simulink library "FireflySimLib"  (R2018a)
settings: Solver=VariableStepAuto  StartTime=0.0  StopTime=10.0  RelTol=1e-3
values from neighbouring files (symbols this model uses):
  mass = parmodel.mass    [LowLevelGeometricController.m]
  p = [ -lengthsoccerfield(1)/2*(yi-centersoccerfieldpic(2))/centersoccerfieldpic(2) lengthsoccerfield(2)/2*(xi-centersoccerfieldpic(1))/centersoccerfieldpic(2)]    [clicks2traj.m]    (also in lqrtrajgeneration.m = size(M,1))
  T = Tlowerlimit    [LowLevelGeometricController.m]    (also in T.mat = ; lqrtrajgeneration.m = T-T(1))
undefined symbols (not defined in the file or in its folder): cdrag, g, lambda, mat2cell, omega, parcontroller, pose0, v
libraries: vrlib x5, sharedtransform x3, dspindex x1, dspsigattribs x1, shared6dof x1
settings Model: Creator=duarteantunes  LastModifiedBy=duarteantunes

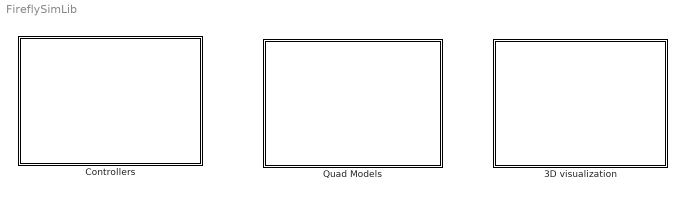
== system FireflySimLib ==
  3D visualization : Subsystem
      mask Display: image('/Users/duarteantunes/surfdrive/AssistantProfessor/Software/Matlab/Firefly/tests/FirstProject/RobotLove/Aux/showpic.png');
  Controllers : Subsystem
      mask Display: image('/Users/duarteantunes/surfdrive/AssistantProfessor/Software/Matlab/Firefly/tests/FirstProject/RobotLove/Aux/pid.png');
  Quad Models : Subsystem
      mask Display: image('/Users/duarteantunes/surfdrive/AssistantProfessor/Software/Matlab/Firefly/tests/FirstProject/RobotLove/Aux/drone.jpg');

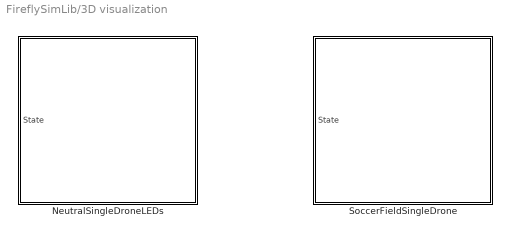
== system FireflySimLib/3D visualization ==
  NeutralSingleDroneLEDs : Subsystem
  SoccerFieldSingleDrone : Subsystem  AncestorBlock=FireflyLib/3D visualization/NeutralSingleDroneLEDs

== system FireflySimLib/Controllers ==
  Controller : Subsystem

== system FireflySimLib/Quad Models ==
  Quad rigid body model : Subsystem

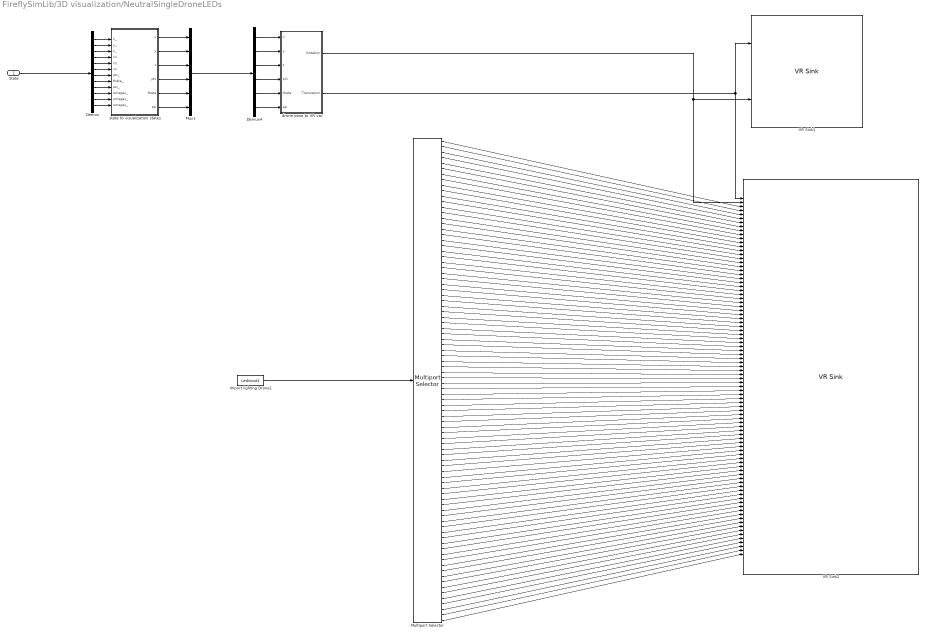
== system FireflySimLib/3D visualization/NeutralSingleDroneLEDs ==
  State : Inport
  Demux : Demux  Outputs=12
  Demux4 : Demux  Outputs=6
  Import lighting Drone1 : FromWorkspace  VariableName=Ledinput1  SampleTime=0
  Multiport Selector : dspindex/Multiport Selector  rowsOrCols=Rows  idxCellArray=mat2cell([1:88],1,ones(88,1))  idxErrMode=Clip Index
  Mux1 : Mux  Inputs=6
  VR Sink1 : vrlib/VR Sink  InstantiateOnLoad=on  SampleTime=0.1  ViewEnable=on  RemoteChange=off  RemoteView=off  FieldsWritten=Quad1.translation.3.1.1.double#Quad1.rotation.4.1.1.double  WorldFileName=SoccerFieldSingleDrone.wrl  AutoView=off  VideoDimensions=[]  AllowVariableSize=off
      settings: SourceProductBaseCode=VR
  VR Sink2 : vrlib/VR Sink  InstantiateOnLoad=on  SampleTime=0.1  ViewEnable=on  RemoteChange=off  RemoteView=off  FieldsWritten=Quad1.translation.3.1.1.double#Quad1.rotation.4.1.1.double#led1_1.emissiveColor.3.1.1.double#led1_2.emissiveColor.3.1.1.double#led1_3.emissiveColor.3.1.1.double#led1_4.emissiveColor.3.1.1.double#led1_5.emissiveColor.3.1.1.double#led1_6.emissiveColor.3.1.1.double#led1_7.emissiveColor.3.1.1.double#led1_8.emissiveColor.3.1.1.double#led1_9.emissiveColor.3.1.1.double#led1_10.emissiveColor.3.1.1.double#led1_11.emissiveColor.3.1.1.double#led1_12.emissiveColor.3.1.1.double#led1_13.emissiveColor.3.1.1.double#led1_14.emissiveColor.3.1.1.double#led1_15.emissiveColor.3.1.1.double#led1_16.emissiveColor.3.1.1.double#led1_17.emissiveColor.3.1.1.double#led1_18.emissiveColor.3.1.1.double#led1_19.emissiveColor.3.1.1.double#led1_20.emissiveColor.3.1.1.double#led1_21.emissiveColor.3.1.1.double#led1_22.emissiveColor.3.1.1.double#led1_23.emissiveColor.3.1.1.double#led1_24.emissiveColor.3.1.1.double#led1_25.emissiveColor.3.1.1.double#led1_26.emissiveColor.3.1.1.double#led1_27.emissiveColor.3.1.1.double#led1_28.emissiveColor.3.1.1.double#led1_29.emissiveColor.3.1.1.double#led1_30.emissiveColor.3.1.1.double#led1_31.emissiveColor.3.1.1.double#led1_32.emissiveColor.3.1.1.double#led1_33.emissiveColor.3.1.1.double#led1_34.emissiveColor.3.1.1.double#led1_35.emissiveColor.3.1.1.double#led1_36.emissiveColor.3.1.1.double#led1_37.emissiveColor.3.1.1.double#led1_38.emissiveColor.3.1.1.double#led1_39.emissiveColor.3.1.1.double#led1_40.emissiveColor.3.1.1.double#led1_41.emissiveColor.3.1.1.double#led1_42.emissiveColor.3.1.1.double#led1_43.emissiveColor.3.1.1.double#led1_44.emissiveColor.3.1.1.double#led1_45.emissiveColor.3.1.1.double#led1_46.emissiveColor.3.1.1.double#led1_47.emissiveColor.3.1.1.double#led1_48.emissiveColor.3.1.1.double#led1_49.emissiveColor.3.1.1.double#led1_50.emissiveColor.3.1.1.double#led1_51.emissiveColor.3.1.1.double#led1_52.emissiveColor.3.1.1.double#led1_53.emissiveColor.3.1.1.double#led1_54.emissiveColor.3.1.1.double#led1_55.emissiveColor.3.1.1.double#led1_56.emissiveColor.3.1.1.double#led1_57.emissiveColor.3.1.1.double#led1_58.emissiveColor.3.1.1.double#led1_59.emissiveColor.3.1.1.double#led1_60.emissiveColor.3.1.1.double#led1_61.emissiveColor.3.1.1.double#led1_62.emissiveColor.3.1.1.double#led1_63.emissiveColor.3.1.1.double#led1_64.emissiveColor.3.1.1.double#led1_65.emissiveColor.3.1.1.double#led1_66.emissiveColor.3.1.1.double#led1_67.emissiveColor.3.1.1.double#led1_68.emissiveColor.3.1.1.double#led1_69.emissiveColor.3.1.1.double#led1_70.emissiveColor.3.1.1.double#led1_71.emissiveColor.3.1.1.double#led1_72.emissiveColor.3.1.1.double#led1_73.emissiveColor.3.1.1.double#led1_74.emissiveColor.3.1.1.double#led1_75.emissiveColor.3.1.1.double#led1_76.emissiveColor.3.1.1.double#led1_77.emissiveColor.3.1.1.double#led1_78.emissiveColor.3.1.1.double#led1_79.emissiveColor.3.1.1.double#led1_80.emissiveColor.3.1.1.double#led1_81.emissiveColor.3.1.1.double#led1_82.emissiveColor.3.1.1.double#led1_83.emissiveColor.3.1.1.double#led1_84.emissiveColor.3.1.1.double#led1_85.emissiveColor.3.1.1.double#led1_86.emissiveColor.3.1.1.double#led1_87.emissiveColor.3.1.1.double#led1_88.emissiveColor.3.1.1.double  WorldFileName=NeutralSingleDroneLEDs.wrl  AutoView=off  VideoDimensions=[]  AllowVariableSize=off
      settings: SourceProductBaseCode=VR
  drone pose to VR var : Subsystem
  state to visualization states : Subsystem
  wires:
  Demux/2 -> state to visualization states/2(y_)
  Demux/9 -> state to visualization states/9(psi_)
  State/1 -> Demux/1
  Demux/11 -> state to visualization states/11(omegay_)
  Demux/10 -> state to visualization states/10(omegax_)
  Demux/12 -> state to visualization states/12(omegaz_)
  Demux/1 -> state to visualization states/1(x_)
  Demux/4 -> state to visualization states/4(vx)
  Demux/8 -> state to visualization states/8(theta_)
  Demux/6 -> state to visualization states/6(vz)
  Demux/3 -> state to visualization states/3(z_)
  Demux/5 -> state to visualization states/5(vy)
  Demux/7 -> state to visualization states/7(phi_)
  drone pose to VR var/2(Translation) -> VR Sink1/1, VR Sink2/1
  Import lighting Drone1/1 -> Multiport Selector/1
  state to visualization states/1(x) -> Mux1/1
  state to visualization states/2(y) -> Mux1/2
  state to visualization states/4(phi) -> Mux1/4
  state to visualization states/3(z) -> Mux1/3
  state to visualization states/6(psi) -> Mux1/6
  state to visualization states/5(theta) -> Mux1/5
  Mux1/1 -> Demux4/1
  Demux4/6 -> drone pose to VR var/6(psi)
  Demux4/5 -> drone pose to VR var/5(theta)
  Demux4/4 -> drone pose to VR var/4(phi)
  Demux4/3 -> drone pose to VR var/3(z)
  Demux4/2 -> drone pose to VR var/2(y)
  Demux4/1 -> drone pose to VR var/1(x)
  drone pose to VR var/1(Rotation) -> VR Sink1/2, VR Sink2/2
  Multiport Selector/88 -> VR Sink2/90
  Multiport Selector/87 -> VR Sink2/89
  Multiport Selector/86 -> VR Sink2/88
  Multiport Selector/85 -> VR Sink2/87
  Multiport Selector/84 -> VR Sink2/86
  Multiport Selector/83 -> VR Sink2/85
  Multiport Selector/82 -> VR Sink2/84
  Multiport Selector/80 -> VR Sink2/82
  Multiport Selector/81 -> VR Sink2/83
  Multiport Selector/79 -> VR Sink2/81
  Multiport Selector/78 -> VR Sink2/80
  Multiport Selector/77 -> VR Sink2/79
  Multiport Selector/76 -> VR Sink2/78
  Multiport Selector/75 -> VR Sink2/77
  Multiport Selector/74 -> VR Sink2/76
  Multiport Selector/73 -> VR Sink2/75
  Multiport Selector/72 -> VR Sink2/74
  Multiport Selector/71 -> VR Sink2/73
  Multiport Selector/69 -> VR Sink2/71
  Multiport Selector/70 -> VR Sink2/72
  Multiport Selector/68 -> VR Sink2/70
  Multiport Selector/66 -> VR Sink2/68
  Multiport Selector/67 -> VR Sink2/69
  Multiport Selector/65 -> VR Sink2/67
  Multiport Selector/63 -> VR Sink2/65
  Multiport Selector/64 -> VR Sink2/66
  Multiport Selector/62 -> VR Sink2/64
  Multiport Selector/61 -> VR Sink2/63
  Multiport Selector/60 -> VR Sink2/62
  Multiport Selector/59 -> VR Sink2/61
  Multiport Selector/58 -> VR Sink2/60
  Multiport Selector/57 -> VR Sink2/59
  Multiport Selector/55 -> VR Sink2/57
  Multiport Selector/56 -> VR Sink2/58
  Multiport Selector/54 -> VR Sink2/56
  Multiport Selector/53 -> VR Sink2/55
  Multiport Selector/52 -> VR Sink2/54
  Multiport Selector/51 -> VR Sink2/53
  Multiport Selector/50 -> VR Sink2/52
  Multiport Selector/49 -> VR Sink2/51
  Multiport Selector/48 -> VR Sink2/50
  Multiport Selector/47 -> VR Sink2/49
  Multiport Selector/46 -> VR Sink2/48
  Multiport Selector/45 -> VR Sink2/47
  Multiport Selector/43 -> VR Sink2/45
  Multiport Selector/44 -> VR Sink2/46
  Multiport Selector/42 -> VR Sink2/44
  Multiport Selector/41 -> VR Sink2/43
  Multiport Selector/37 -> VR Sink2/39
  Multiport Selector/35 -> VR Sink2/37
  Multiport Selector/33 -> VR Sink2/35
  Multiport Selector/31 -> VR Sink2/33
  Multiport Selector/30 -> VR Sink2/32
  Multiport Selector/28 -> VR Sink2/30
  Multiport Selector/24 -> VR Sink2/26
  Multiport Selector/22 -> VR Sink2/24
  Multiport Selector/26 -> VR Sink2/28
  Multiport Selector/25 -> VR Sink2/27
  Multiport Selector/20 -> VR Sink2/22
  Multiport Selector/23 -> VR Sink2/25
  Multiport Selector/21 -> VR Sink2/23
  Multiport Selector/19 -> VR Sink2/21
  Multiport Selector/18 -> VR Sink2/20
  Multiport Selector/17 -> VR Sink2/19
  Multiport Selector/16 -> VR Sink2/18
  Multiport Selector/27 -> VR Sink2/29
  Multiport Selector/29 -> VR Sink2/31
  Multiport Selector/32 -> VR Sink2/34
  Multiport Selector/34 -> VR Sink2/36
  Multiport Selector/36 -> VR Sink2/38
  Multiport Selector/38 -> VR Sink2/40
  Multiport Selector/39 -> VR Sink2/41
  Multiport Selector/40 -> VR Sink2/42
  Multiport Selector/15 -> VR Sink2/17
  Multiport Selector/14 -> VR Sink2/16
  Multiport Selector/13 -> VR Sink2/15
  Multiport Selector/12 -> VR Sink2/14
  Multiport Selector/11 -> VR Sink2/13
  Multiport Selector/10 -> VR Sink2/12
  Multiport Selector/9 -> VR Sink2/11
  Multiport Selector/7 -> VR Sink2/9
  Multiport Selector/8 -> VR Sink2/10
  Multiport Selector/6 -> VR Sink2/8
  Multiport Selector/4 -> VR Sink2/6
  Multiport Selector/5 -> VR Sink2/7
  Multiport Selector/3 -> VR Sink2/5
  Multiport Selector/2 -> VR Sink2/4
  Multiport Selector/1 -> VR Sink2/3

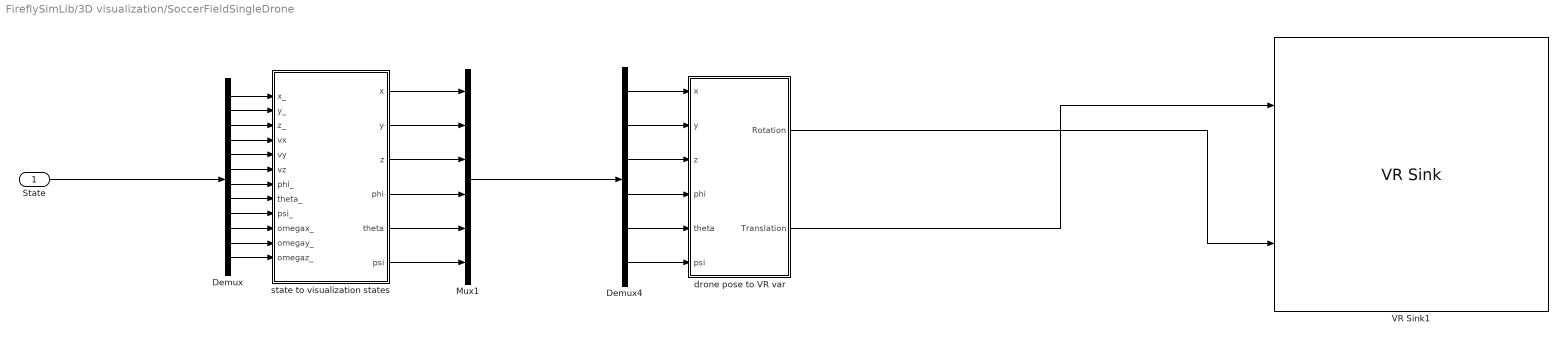
== system FireflySimLib/3D visualization/SoccerFieldSingleDrone ==
  State : Inport
  Demux : Demux  Outputs=12
  Demux4 : Demux  Outputs=6
  Mux1 : Mux  Inputs=6
  VR Sink1 : vrlib/VR Sink  InstantiateOnLoad=on  SampleTime=0.1  ViewEnable=on  RemoteChange=off  RemoteView=off  FieldsWritten=Quad1.translation.3.1.1.double#Quad1.rotation.4.1.1.double  WorldFileName=SoccerFieldSingleDrone.wrl  AutoView=off  VideoDimensions=[]  AllowVariableSize=off
      settings: SourceProductBaseCode=VR
  drone pose to VR var : Subsystem
  state to visualization states : Subsystem
  wires:
  Demux/2 -> state to visualization states/2(y_)
  Demux/9 -> state to visualization states/9(psi_)
  State/1 -> Demux/1
  Demux/11 -> state to visualization states/11(omegay_)
  Demux/10 -> state to visualization states/10(omegax_)
  Demux/12 -> state to visualization states/12(omegaz_)
  Demux/1 -> state to visualization states/1(x_)
  Demux/4 -> state to visualization states/4(vx)
  Demux/8 -> state to visualization states/8(theta_)
  Demux/6 -> state to visualization states/6(vz)
  Demux/3 -> state to visualization states/3(z_)
  Demux/5 -> state to visualization states/5(vy)
  Demux/7 -> state to visualization states/7(phi_)
  drone pose to VR var/2(Translation) -> VR Sink1/1
  state to visualization states/1(x) -> Mux1/1
  state to visualization states/2(y) -> Mux1/2
  state to visualization states/4(phi) -> Mux1/4
  state to visualization states/3(z) -> Mux1/3
  state to visualization states/6(psi) -> Mux1/6
  state to visualization states/5(theta) -> Mux1/5
  Mux1/1 -> Demux4/1
  Demux4/6 -> drone pose to VR var/6(psi)
  Demux4/5 -> drone pose to VR var/5(theta)
  Demux4/4 -> drone pose to VR var/4(phi)
  Demux4/3 -> drone pose to VR var/3(z)
  Demux4/2 -> drone pose to VR var/2(y)
  Demux4/1 -> drone pose to VR var/1(x)
  drone pose to VR var/1(Rotation) -> VR Sink1/2

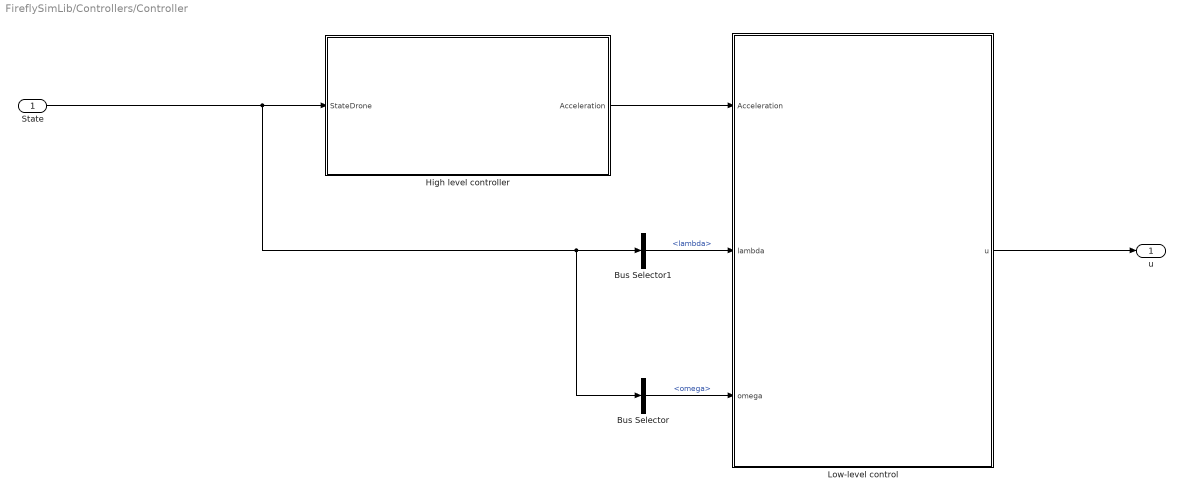
== system FireflySimLib/Controllers/Controller ==
  State : Inport
  Bus Selector : BusSelector  OutputSignals=omega
  Bus Selector1 : BusSelector  OutputSignals=lambda
  High level controller : Subsystem
  Low-level control : Subsystem
  u : Outport
  wires:
  High level controller/1(Acceleration) -> Low-level control/1(Acceleration)
  Bus Selector/1 -> Low-level control/3(omega)  "<omega>"
  Bus Selector1/1 -> Low-level control/2(lambda)  "<lambda>"
  State/1 -> Bus Selector/1, Bus Selector1/1, High level controller/1(StateDrone)
  Low-level control/1(u) -> u/1

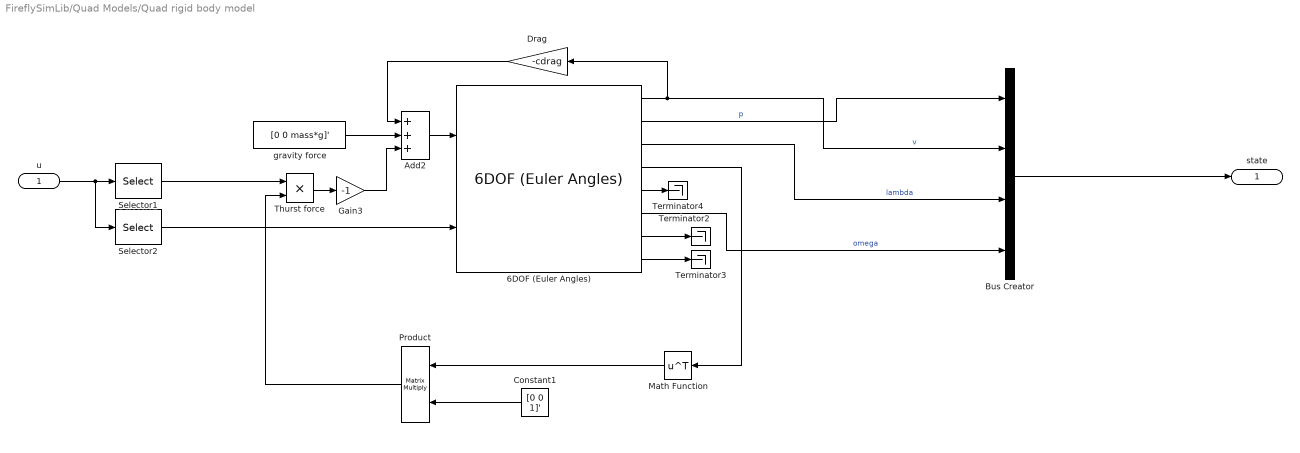
== system FireflySimLib/Quad Models/Quad rigid body model ==
  "u " : Inport
  6DOF (Euler Angles) : shared6dof/6DOF (Euler Angles)  units=Metric (MKS)  mtype=Fixed  rep=Euler Angles  xme_0=pose0(1:3)  Vm_0=[0 0 0]  eul_0=[0 0 pose0(4)]  pm_0=[0 0 0]  mass_0=mass  mass_e=0.5  mass_f=2.0  inertia=MomInertia  inertia_e=eye(3)  inertia_f=2*eye(3)  k_quat=1.0  vre_flag=on  abi_flag=off  aMode=aMode
      settings: SourceProductBaseCode=AE
  Add2 : Sum  Inputs=+++
  Bus Creator : BusCreator  Inputs=p,v,lambda,omega
  Constant1 : Constant  Value=[0 0 1]'
  Drag : Gain  Gain=-cdrag
  Gain3 : Gain  Gain=-1
  Math Function : Math  Operator=transpose  SaturateOnIntegerOverflow=on
  Product : Product  Multiplication=Matrix(*)
  Selector1 : Selector  InputPortWidth=4  IndexOptions=Index vector (dialog)  Indices=1  OutputSizes=1
  Selector2 : Selector  InputPortWidth=4  IndexOptions=Index vector (dialog)  Indices=[2,3,4]  OutputSizes=1
  Terminator2 : Terminator
  Terminator3 : Terminator
  Terminator4 : Terminator
  Thurst force : Product
  gravity force : Constant  Value=[0 0 mass*g]'  VectorParams1D=off
  state : Outport
  wires:
  Constant1/1 -> Product/2
  Add2/1 -> 6DOF (Euler Angles)/1
  Math Function/1 -> Product/1
  Product/1 -> Thurst force/2
  6DOF (Euler Angles)/1 -> Drag/1, Bus Creator/2  "v"
  6DOF (Euler Angles)/7 -> Terminator2/1
  6DOF (Euler Angles)/8 -> Terminator3/1
  6DOF (Euler Angles)/5 -> Terminator4/1
  Thurst force/1 -> Gain3/1
  gravity force/1 -> Add2/2
  Drag/1 -> Add2/1
  Gain3/1 -> Add2/3
  6DOF (Euler Angles)/4 -> Math Function/1
  Bus Creator/1 -> state/1
  6DOF (Euler Angles)/6 -> Bus Creator/4  "omega"
  6DOF (Euler Angles)/3 -> Bus Creator/3  "lambda"
  6DOF (Euler Angles)/2 -> Bus Creator/1  "p"
  "u "/1 -> Selector2/1, Selector1/1
  Selector1/1 -> Thurst force/1
  Selector2/1 -> 6DOF (Euler Angles)/2

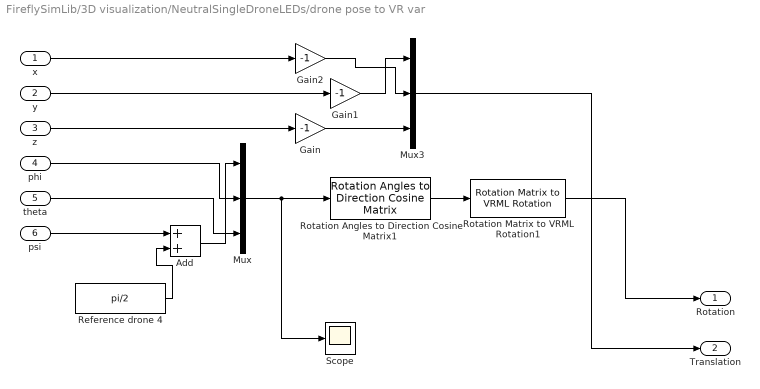
== system FireflySimLib/3D visualization/NeutralSingleDroneLEDs/drone pose to VR var ==
  x : Inport
  y : Inport  Port=2
  z : Inport  Port=3
  phi : Inport  Port=4
  theta : Inport  Port=5
  psi : Inport  Port=6
  Add : Sum
  Gain : Gain  Gain=-1
  Gain1 : Gain  Gain=-1
  Gain2 : Gain  Gain=-1
  Mux : Mux  Inputs=3
  Mux3 : Mux  Inputs=3
  Reference drone 4 : Constant  Value=pi/2
  Rotation Angles to Direction Cosine Matrix1 : sharedtransform/Rotation Angles to Direction Cosine Matrix  rotationOrder=ZYX  aMode=aMode
      settings: SourceProductBaseCode=AE
  Rotation Matrix to VRML Rotation1 : vrlib/Utilities/Rotation Matrix to VRML Rotation  maxzero=1e-12
      settings: SourceProductName=Simulink 3D Animation  SourceProductBaseCode=VR
  Scope : Scope
  Rotation : Outport
  Translation : Outport  Port=2
  wires:
  theta/1 -> Mux/3
  phi/1 -> Mux/2
  Gain/1 -> Mux3/3
  Gain1/1 -> Mux3/1
  z/1 -> Gain/1
  Gain2/1 -> Mux3/2
  x/1 -> Gain2/1
  y/1 -> Gain1/1
  Mux/1 -> Rotation Angles to Direction Cosine Matrix1/1, Scope/1
  Rotation Angles to Direction Cosine Matrix1/1 -> Rotation Matrix to VRML Rotation1/1
  psi/1 -> Add/1
  Reference drone 4/1 -> Add/2
  Add/1 -> Mux/1
  Mux3/1 -> Translation/1
  Rotation Matrix to VRML Rotation1/1 -> Rotation/1

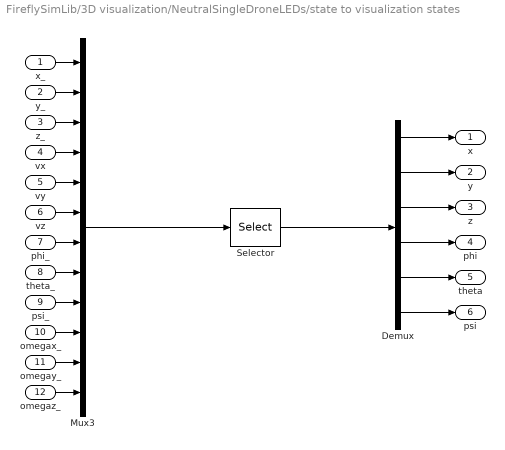
== system FireflySimLib/3D visualization/NeutralSingleDroneLEDs/state to visualization states ==
  x_ : Inport
  y_ : Inport  Port=2
  z_ : Inport  Port=3
  vx : Inport  Port=4
  vy : Inport  Port=5
  vz : Inport  Port=6
  phi_ : Inport  Port=7
  theta_ : Inport  Port=8
  psi_ : Inport  Port=9
  omegax_ : Inport  Port=10
  omegay_ : Inport  Port=11
  omegaz_ : Inport  Port=12
  Demux : Demux  Outputs=6
  Mux3 : Mux  Inputs=12
  Selector : Selector  InputPortWidth=12  IndexOptions=Index vector (dialog)  Indices=[1,2,3,7,8,9]  OutputSizes=1
  x : Outport
  y : Outport  Port=2
  z : Outport  Port=3
  phi : Outport  Port=4
  theta : Outport  Port=5
  psi : Outport  Port=6
  wires:
  Selector/1 -> Demux/1
  Mux3/1 -> Selector/1
  Demux/1 -> x/1
  Demux/2 -> y/1
  Demux/3 -> z/1
  Demux/4 -> phi/1
  Demux/5 -> theta/1
  Demux/6 -> psi/1
  z_/1 -> Mux3/3
  vy/1 -> Mux3/5
  x_/1 -> Mux3/1
  y_/1 -> Mux3/2
  vx/1 -> Mux3/4
  vz/1 -> Mux3/6
  phi_/1 -> Mux3/7
  omegax_/1 -> Mux3/10
  theta_/1 -> Mux3/8
  psi_/1 -> Mux3/9
  omegay_/1 -> Mux3/11
  omegaz_/1 -> Mux3/12

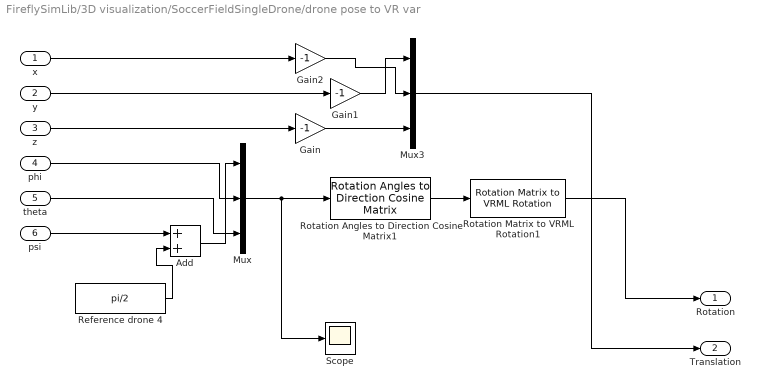
== system FireflySimLib/3D visualization/SoccerFieldSingleDrone/drone pose to VR var ==
  x : Inport
  y : Inport  Port=2
  z : Inport  Port=3
  phi : Inport  Port=4
  theta : Inport  Port=5
  psi : Inport  Port=6
  Add : Sum
  Gain : Gain  Gain=-1
  Gain1 : Gain  Gain=-1
  Gain2 : Gain  Gain=-1
  Mux : Mux  Inputs=3
  Mux3 : Mux  Inputs=3
  Reference drone 4 : Constant  Value=pi/2
  Rotation Angles to Direction Cosine Matrix1 : sharedtransform/Rotation Angles to Direction Cosine Matrix  rotationOrder=ZYX  aMode=aMode
      settings: SourceProductBaseCode=AE
  Rotation Matrix to VRML Rotation1 : vrlib/Utilities/Rotation Matrix to VRML Rotation  maxzero=1e-12
      settings: SourceProductName=Simulink 3D Animation  SourceProductBaseCode=VR
  Scope : Scope
  Rotation : Outport
  Translation : Outport  Port=2
  wires:
  theta/1 -> Mux/3
  phi/1 -> Mux/2
  Gain/1 -> Mux3/3
  Gain1/1 -> Mux3/1
  z/1 -> Gain/1
  Gain2/1 -> Mux3/2
  x/1 -> Gain2/1
  y/1 -> Gain1/1
  Mux/1 -> Rotation Angles to Direction Cosine Matrix1/1, Scope/1
  Rotation Angles to Direction Cosine Matrix1/1 -> Rotation Matrix to VRML Rotation1/1
  psi/1 -> Add/1
  Reference drone 4/1 -> Add/2
  Add/1 -> Mux/1
  Mux3/1 -> Translation/1
  Rotation Matrix to VRML Rotation1/1 -> Rotation/1

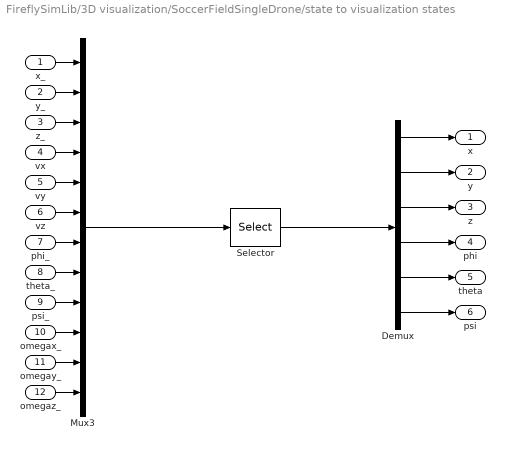
== system FireflySimLib/3D visualization/SoccerFieldSingleDrone/state to visualization states ==
  x_ : Inport
  y_ : Inport  Port=2
  z_ : Inport  Port=3
  vx : Inport  Port=4
  vy : Inport  Port=5
  vz : Inport  Port=6
  phi_ : Inport  Port=7
  theta_ : Inport  Port=8
  psi_ : Inport  Port=9
  omegax_ : Inport  Port=10
  omegay_ : Inport  Port=11
  omegaz_ : Inport  Port=12
  Demux : Demux  Outputs=6
  Mux3 : Mux  Inputs=12
  Selector : Selector  InputPortWidth=12  IndexOptions=Index vector (dialog)  Indices=[1,2,3,7,8,9]  OutputSizes=1
  x : Outport
  y : Outport  Port=2
  z : Outport  Port=3
  phi : Outport  Port=4
  theta : Outport  Port=5
  psi : Outport  Port=6
  wires:
  Selector/1 -> Demux/1
  Mux3/1 -> Selector/1
  Demux/1 -> x/1
  Demux/2 -> y/1
  Demux/3 -> z/1
  Demux/4 -> phi/1
  Demux/5 -> theta/1
  Demux/6 -> psi/1
  z_/1 -> Mux3/3
  vy/1 -> Mux3/5
  x_/1 -> Mux3/1
  y_/1 -> Mux3/2
  vx/1 -> Mux3/4
  vz/1 -> Mux3/6
  phi_/1 -> Mux3/7
  omegax_/1 -> Mux3/10
  theta_/1 -> Mux3/8
  psi_/1 -> Mux3/9
  omegay_/1 -> Mux3/11
  omegaz_/1 -> Mux3/12

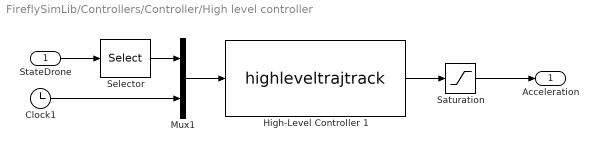
== system FireflySimLib/Controllers/Controller/High level controller ==
  StateDrone : Inport
  Clock1 : Clock
  High-Level Controller 1 : S-Function  FunctionName=highleveltrajtrack  Parameters=T,parcontroller  SFunctionDeploymentMode=off  EnableBusSupport=off
  Mux1 : Mux  Inputs=2
  Saturation : Saturate  UpperLimit=10  LowerLimit=-10
  Selector : Selector  InputPortWidth=12  IndexOptions=Index vector (dialog)  Indices=[1,2,3,9,4,5,6,12]  OutputSizes=1
  Acceleration : Outport
  wires:
  StateDrone/1 -> Selector/1
  Clock1/1 -> Mux1/2
  High-Level Controller 1/1 -> Saturation/1
  Saturation/1 -> Acceleration/1
  Mux1/1 -> High-Level Controller 1/1
  Selector/1 -> Mux1/1

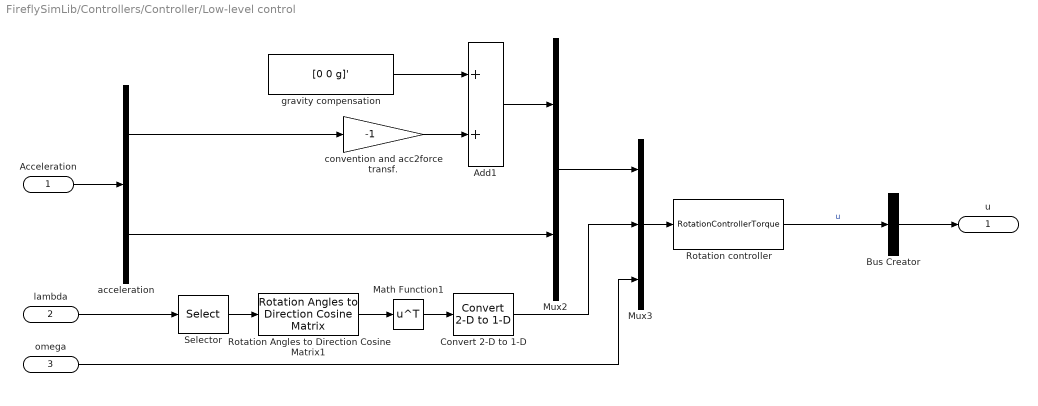
== system FireflySimLib/Controllers/Controller/Low-level control ==
  Acceleration : Inport
  lambda : Inport  Port=2
  omega : Inport  Port=3
  Add1 : Sum
  Bus Creator : BusCreator  Inputs=1
  Convert 2-D to 1-D : dspsigattribs/Convert 2-D to 1-D
      settings: SourceProductName=DSP System Toolbox  SourceProductBaseCode=DS
  Math Function1 : Math  Operator=transpose  SaturateOnIntegerOverflow=on
  Mux2 : Mux  Inputs=2
  Mux3 : Mux  Inputs=3
  Rotation Angles to Direction Cosine Matrix1 : sharedtransform/Rotation Angles to Direction Cosine Matrix  rotationOrder=ZYX  aMode=aMode
      settings: SourceProductBaseCode=AE
  Rotation controller : S-Function  FunctionName=RotationControllerTorque  Parameters=mass,MomInertia, parcontroller  SFunctionDeploymentMode=off  EnableBusSupport=off
  Selector : Selector  InputPortWidth=3  IndexOptions=Index vector (dialog)  Indices=[3,2,1]  OutputSizes=1
  acceleration : Demux  Outputs=[3,1]
  convention and acc2force transf. : Gain  Gain=-1
  gravity compensation : Constant  Value=[0 0 g]'  VectorParams1D=off
  u : Outport
  wires:
  convention and acc2force transf./1 -> Add1/2
  Add1/1 -> Mux2/1
  Mux2/1 -> Mux3/1
  gravity compensation/1 -> Add1/1
  acceleration/1 -> convention and acc2force transf./1
  Mux3/1 -> Rotation controller/1
  omega/1 -> Mux3/3
  Acceleration/1 -> acceleration/1
  acceleration/2 -> Mux2/2
  Math Function1/1 -> Convert 2-D to 1-D/1
  Convert 2-D to 1-D/1 -> Mux3/2
  Rotation Angles to Direction Cosine Matrix1/1 -> Math Function1/1
  Selector/1 -> Rotation Angles to Direction Cosine Matrix1/1
  lambda/1 -> Selector/1
  Rotation controller/1 -> Bus Creator/1  "u"
  Bus Creator/1 -> u/1
